simulink model "ExoskeletonControlModel"  (R2022b)
settings: Solver=ode3  StartTime=0.0  StopTime=inf  FixedStep=Ts  RelTol=1e-3
PreLoadFcn:
  | Ts_IO204 = 0.001;
  | 
  | if ~exist('Ts', 'var')
  | Ts = 0.001;
  | end
  | if ~exist('FPGA_Frequency', 'var')
  | FPGA_Frequency = 75000000;
  | end
  | 
  | ts_IO612 = 1e-3;
  | 
  | load('TargetReached.mat')
  | load('ActualPos_inc.mat')
model workspace (MAT data in the model file):
  DeltaData : timeseries (value not decoded)
  EC45_deg2incs = 2276
  EC60_deg2inc = 5461
  EC90_deg2incs = 7111
  Enc2rad_18bit = 2.3968e-05
  Enc2rad_19bit = 1.1984e-05
  Enc2rad_20bit = 5.9921e-06
  GiulioModel : robotics.RigidBodyTree (value not decoded)
  Giulio_Spheric_model : robotics.RigidBodyTree (value not decoded)
  Offset1_ticks = 571315
  Offset2_ticks = 590938.9928
  Offset3_ticks = 457912.8279
  Offset4_ticks = 482293.9763
  Offset5_ticks = 598735.9316
  Offset_M1 = 1.12645499896
  Offset_M2 = 4.02728553608
  Offset_M3 = 5.48587511336
  Offset_M4 = 2.03717511516
  Offset_M5 = 4.4996674016
  T1_Nm : object (value not decoded)
  T2_Nm : object (value not decoded)
  TBmodel : robotics.RigidBodyTree (value not decoded)
  Ts = 0.002
  Xg : object (value not decoded)
  Yg : object (value not decoded)
  Zg : object (value not decoded)
  a2 = 0.27
  change_variable = 0
  d1 = [0 0 0 0 0 0 0 0 0 0 0 0 ... (30001 elements, 30001x1)]
  d1_1 = 0.21074
  d2 = [0 0 0 0 0 0 0 0 0 0 0 0 ... (30001 elements, 30001x1)]
  d2_1 = 0.04864
  d3 = [0 0 0 0 0 0 0 0 0 0 0 0 ... (30001 elements, 30001x1)]
  d4 = [0 0 0 0 0 0 0 0 0 0 0 0 ... (30001 elements, 30001x1)]
  d5 = [0 0 0 0 0 0 0 0 0 0 0 0 ... (30001 elements, 30001x1)]
  d6 = [0 0 0 0 0 0 0 0 0 0 0 0 ... (30001 elements, 30001x1)]
  ee_x = -0.2852
  ee_y = -0.3683
  ee_z = -0.0386
  enc2rad_EC45 = 7.6699e-06
  enc2rad_EC90 = 2.3969e-05
  k1_Nm_ticks = 0.00923
  k2_Nm_ticks = 0.0257
  k3_Nm_ticks = 0.00692
  k4_Nm_ticks = 0.00729
  k5_Nm_ticks = 0.00641
  lower_lim_m1 = -330000
  lower_lim_m2 = -235302
  lower_lim_m3 = -132865
  lower_lim_m4 = -152732
  lower_lim_m5 = -138363
  lower_lim_m6 = -200325
  m1 = 2.441408578
  m2 = 3.750007
  m3 = 1.56250298
  m4 = 1.56250298
  m5 = 1.56250298
  m6 = 1.56250298
  n_oversampling = 8
  offset_sea_1 = 0.5547
  offset_sea_2 = 2.8595
  offset_sea_3 = 3.5058
  offset_sea_4 = 2.8586
  offset_sea_5 = 2.8736
  params : AKSIM (value not decoded)
  pos_th_neg = -180000
  pos_th_pos = 180000
  q1 = -1819347
  q2 = -196752
  q3 = -596465
  q4 = -556807
  q5 = -573932
  q6 = -489063
  sine = [0 0.187999937334 0.751998997352 1.69199492401 3.0079839574 4.6999608335 6.76791878442 9.21184953835 12.0317433196 15.2275888485 18.7993733417 22.7470825122 ... (12501 elements, 12501x1)]
  start : object (value not decoded)
  switch_admittance = 1
  t1 : object (value not decoded)
  t2 : object (value not decoded)
  torsionalStiffnes_M1 = 384.88
  torsionalStiffnes_M2 = 1500
  torsionalStiffnes_M3 = 901.97
  torsionalStiffnes_M4 = 950.86
  torsionalStiffnes_M5 = 930
  torsionalStiffnes_M6 = 914
  upper_lim_m1 = 340000
  upper_lim_m2 = 95467
  upper_lim_m3 = 164951
  upper_lim_m4 = 210607
  upper_lim_m5 = 252595
  upper_lim_m6 = 96694
  vel_th_neg = -100
  vel_th_pos = 100
  x = 0
undefined symbols (not defined in the file): C, DiscIntNeverNeededParam
libraries: canmsglib x285, speedgoatlib_IO614 x245, simulink x26, slrealtimeloglib x9, simulink_extras x6, robotmaniplib x6
(part 2 of 13)

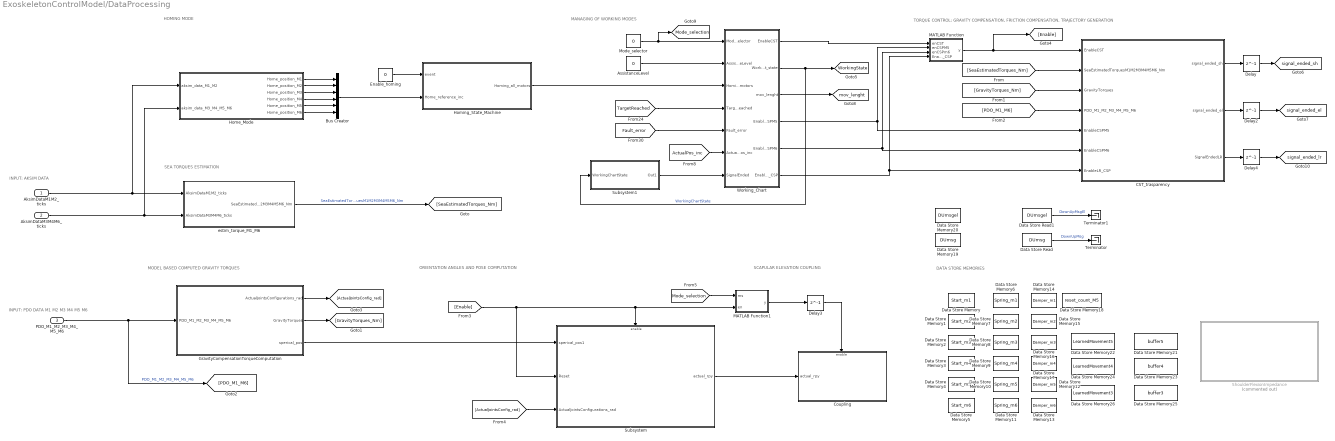
== system ExoskeletonControlModel/DataProcessing ==
  note: SCAPULAR ELEVATION COUPLING
  note: ORIENTATION ANGLES AND POSE COMPUTATION
  note: TORQUE CONTROL: GRAVITY COMPENSATION, FRICTION COMPENSATION, TRAJECTORY GENERATION
  note: MANAGING OF WORKING MODES
  note: DATA STORE MEMORIES
  note: INPUT: AKSIM DATA
  note: HOMING MODE
  note: MODEL BASED COMPUTED GRAVITY TORQUES
  note: INPUT: PDO DATA M1 M2 M3 M4 M5 M6
  note: SEA TORQUES ESTIMATION
  AksimDataM1M2_ticks : Inport
  AksimDataM3M4M6_ticks : Inport  Port=2
  PDO_M1_M2_M3_M4_M5_M6 : Inport  Port=3
  AssistanceLevel : Constant  Value=0
  Bus Creator : BusCreator  Inputs=6
  CST_trasparency : Subsystem
  Coupling : Subsystem
  Data Store Memory18 : DataStoreMemory  DataStoreName=reset_count_M5  ReadBeforeWriteMsg=warning  WriteAfterWriteMsg=warning  WriteAfterReadMsg=warning  ShowAdditionalParam=off  OutDataTypeStr=double
  Data Store Memory21 : DataStoreMemory  DataStoreName=buffer5  ReadBeforeWriteMsg=warning  WriteAfterWriteMsg=warning  WriteAfterReadMsg=warning  ShareAcrossModelInstances=on  VectorParams1D=off  ShowAdditionalParam=off  OutDataTypeStr=double  Dimensions=[10000,1]
  Data Store Memory22 : DataStoreMemory  DataStoreName=LearnedMovement5  ReadBeforeWriteMsg=warning  WriteAfterWriteMsg=warning  WriteAfterReadMsg=warning  ShareAcrossModelInstances=on  VectorParams1D=off  ShowAdditionalParam=off  OutDataTypeStr=double  Dimensions=[10000,1]
  Data Store Memory23 : DataStoreMemory  DataStoreName=buffer4  ReadBeforeWriteMsg=warning  WriteAfterWriteMsg=warning  WriteAfterReadMsg=warning  ShareAcrossModelInstances=on  VectorParams1D=off  ShowAdditionalParam=off  OutDataTypeStr=double  Dimensions=[10000,1]
  Data Store Memory24 : DataStoreMemory  DataStoreName=LearnedMovement4  ReadBeforeWriteMsg=warning  WriteAfterWriteMsg=warning  WriteAfterReadMsg=warning  ShareAcrossModelInstances=on  VectorParams1D=off  ShowAdditionalParam=off  OutDataTypeStr=double  Dimensions=[10000,1]
  Data Store Memory25 : DataStoreMemory  DataStoreName=buffer3  ReadBeforeWriteMsg=warning  WriteAfterWriteMsg=warning  WriteAfterReadMsg=warning  ShareAcrossModelInstances=on  VectorParams1D=off  ShowAdditionalParam=off  OutDataTypeStr=double  Dimensions=[10000,1]
  Data Store Memory26 : DataStoreMemory  DataStoreName=LearnedMovement3  ReadBeforeWriteMsg=warning  WriteAfterWriteMsg=warning  WriteAfterReadMsg=warning  ShareAcrossModelInstances=on  VectorParams1D=off  ShowAdditionalParam=off  OutDataTypeStr=double  Dimensions=[10000,1]
  Data Store Read : DataStoreRead  DataStoreName=DUmsg  IndexOptions=Index vector (dialog)  Indices=1  OutputSizes=1
  Data Store Read1 : DataStoreRead  DataStoreName=DUmsgel  IndexOptions=Index vector (dialog)  Indices=1  OutputSizes=1
  Data Store Memory : DataStoreMemory  DataStoreName=Start_m1  ReadBeforeWriteMsg=warning  WriteAfterWriteMsg=warning  WriteAfterReadMsg=warning  ShowAdditionalParam=off  OutDataTypeStr=double
  Data Store Memory1 : DataStoreMemory  DataStoreName=Start_m2  ReadBeforeWriteMsg=warning  WriteAfterWriteMsg=warning  WriteAfterReadMsg=warning  ShowAdditionalParam=off  OutDataTypeStr=double
  Data Store Memory10 : DataStoreMemory  DataStoreName=Spring_m5  ReadBeforeWriteMsg=warning  WriteAfterWriteMsg=warning  WriteAfterReadMsg=warning  ShowAdditionalParam=off  OutDataTypeStr=double
  Data Store Memory11 : DataStoreMemory  DataStoreName=Spring_m6  ReadBeforeWriteMsg=warning  WriteAfterWriteMsg=warning  WriteAfterReadMsg=warning  ShowAdditionalParam=off  OutDataTypeStr=double
  Data Store Memory12 : DataStoreMemory  DataStoreName=Damper_m5  ReadBeforeWriteMsg=warning  WriteAfterWriteMsg=warning  WriteAfterReadMsg=warning  ShowAdditionalParam=off  OutDataTypeStr=double
  Data Store Memory13 : DataStoreMemory  DataStoreName=Damper_m6  ReadBeforeWriteMsg=warning  WriteAfterWriteMsg=warning  WriteAfterReadMsg=warning  ShowAdditionalParam=off  OutDataTypeStr=double
  Data Store Memory14 : DataStoreMemory  DataStoreName=Damper_m1  ReadBeforeWriteMsg=warning  WriteAfterWriteMsg=warning  WriteAfterReadMsg=warning  ShowAdditionalParam=off  OutDataTypeStr=double
  Data Store Memory15 : DataStoreMemory  DataStoreName=Damper_m2  ReadBeforeWriteMsg=warning  WriteAfterWriteMsg=warning  WriteAfterReadMsg=warning  ShowAdditionalParam=off  OutDataTypeStr=double
  Data Store Memory16 : DataStoreMemory  DataStoreName=Damper_m3  ReadBeforeWriteMsg=warning  WriteAfterWriteMsg=warning  WriteAfterReadMsg=warning  ShowAdditionalParam=off  OutDataTypeStr=double
  Data Store Memory17 : DataStoreMemory  DataStoreName=Damper_m4  ReadBeforeWriteMsg=warning  WriteAfterWriteMsg=warning  WriteAfterReadMsg=warning  ShowAdditionalParam=off  OutDataTypeStr=double
  Data Store Memory19 : DataStoreMemory  DataStoreName=DUmsg  ReadBeforeWriteMsg=warning  WriteAfterWriteMsg=warning  WriteAfterReadMsg=warning  ShowAdditionalParam=off  OutDataTypeStr=double
  Data Store Memory2 : DataStoreMemory  DataStoreName=Start_m3  ReadBeforeWriteMsg=warning  WriteAfterWriteMsg=warning  WriteAfterReadMsg=warning  ShowAdditionalParam=off  OutDataTypeStr=double
  Data Store Memory20 : DataStoreMemory  DataStoreName=DUmsgel  ReadBeforeWriteMsg=warning  WriteAfterWriteMsg=warning  WriteAfterReadMsg=warning  ShowAdditionalParam=off  OutDataTypeStr=double
  Data Store Memory3 : DataStoreMemory  DataStoreName=Start_m4  ReadBeforeWriteMsg=warning  WriteAfterWriteMsg=warning  WriteAfterReadMsg=warning  ShowAdditionalParam=off  OutDataTypeStr=double
  Data Store Memory4 : DataStoreMemory  DataStoreName=Start_m5  ReadBeforeWriteMsg=warning  WriteAfterWriteMsg=warning  WriteAfterReadMsg=warning  ShowAdditionalParam=off  OutDataTypeStr=double
  Data Store Memory5 : DataStoreMemory  DataStoreName=Start_m6  ReadBeforeWriteMsg=warning  WriteAfterWriteMsg=warning  WriteAfterReadMsg=warning  ShowAdditionalParam=off  OutDataTypeStr=double
  Data Store Memory6 : DataStoreMemory  DataStoreName=Spring_m1  ReadBeforeWriteMsg=warning  WriteAfterWriteMsg=warning  WriteAfterReadMsg=warning  ShowAdditionalParam=off  OutDataTypeStr=double
  Data Store Memory7 : DataStoreMemory  DataStoreName=Spring_m2  ReadBeforeWriteMsg=warning  WriteAfterWriteMsg=warning  WriteAfterReadMsg=warning  ShowAdditionalParam=off  OutDataTypeStr=double
  Data Store Memory8 : DataStoreMemory  DataStoreName=Spring_m3  ReadBeforeWriteMsg=warning  WriteAfterWriteMsg=warning  WriteAfterReadMsg=warning  ShowAdditionalParam=off  OutDataTypeStr=double
  Data Store Memory9 : DataStoreMemory  DataStoreName=Spring_m4  ReadBeforeWriteMsg=warning  WriteAfterWriteMsg=warning  WriteAfterReadMsg=warning  ShowAdditionalParam=off  OutDataTypeStr=double
  Delay{,2..4} (4 alike) : Delay  DelayLength=1
  Enable_homing : Constant  Value=0
  GravityCompensationTorqueComputation : Subsystem
  Home_Mode : Subsystem
  Homing_State_Machine : Subsystem
  MATLAB Function : MATLAB Function  TreatAsAtomicUnit=on
  MATLAB Function1 : MATLAB Function  TreatAsAtomicUnit=on
  Mode_selector : Constant  Value=0
  ShoulderFlexionImpedance : Subsystem  Commented=on
  Subsystem : Subsystem
  Subsystem1 : Subsystem
  Terminator : Terminator
  Terminator1 : Terminator
  Working_Chart : Stateflow chart  TreatAsAtomicUnit=on
  estim_torque_M1_M6 : Subsystem
  tag scope: Mode_selection=global, WorkingState=global, mov_lenght=global, signal_ended_el=global, signal_ended_lr=global, signal_ended_sh=global
  wires:
  AksimDataM1M2_ticks/1 -> estim_torque_M1_M6/1(AksimDataM1M2_ticks), Home_Mode/1(aksim_data_M1_M2)
  AksimDataM3M4M6_ticks/1 -> Home_Mode/2(aksim_data_M3_M4_M5_M6), estim_torque_M1_M6/2(AksimDataM3M4M6_ticks)
  estim_torque_M1_M6/1(SeaEstimatedTorquesM1M2M3M4M5M6_Nm) -> [SeaEstimatedTorques_Nm]  "SeaEstimatedTorquesM1M2M3M4M5M6_Nm"
  Home_Mode/1(Home_position_M1) -> Bus Creator/1
  Home_Mode/2(Home_position_M2) -> Bus Creator/2
  Home_Mode/3(Home_position_M3) -> Bus Creator/3
  Home_Mode/4(Home_position_M4) -> Bus Creator/4
  Home_Mode/5(Home_position_M5) -> Bus Creator/5
  Bus Creator/1 -> Homing_State_Machine/2(Home_reference_inc)
  Home_Mode/6(Home_position_M6) -> Bus Creator/6
  GravityCompensationTorqueComputation/1(ActualJointsConfigurations_rad) -> [ActualJointsConfig_rad]
  GravityCompensationTorqueComputation/2(GravityTorques) -> [GravityTorques_Nm]
  GravityCompensationTorqueComputation/3(sperical_pos) -> Subsystem/1(sperical_pos1)
  Subsystem/1(actual_rpy) -> Coupling/1(actual_rpy)
  [Enable] -> Subsystem/2(Reset), Subsystem/Enable, MATLAB Function1/2(en)
  PDO_M1_M2_M3_M4_M5_M6/1 -> [PDO_M1_M6], GravityCompensationTorqueComputation/1(PDO_M1_M2_M3_M4_M5_M6)  "PDO_M1_M2_M3_M4_M5_M6"
  Enable_homing/1 -> Homing_State_Machine/1(event)
  Mode_selector/1 -> [Mode_selection], Working_Chart/1(Mode_selector)
  Homing_State_Machine/1(Homing_all_motors) -> Working_Chart/3(Homing_all_motors)
  Working_Chart/1(EnableCST) -> MATLAB Function/1(enCST)
  [SeaEstimatedTorques_Nm] -> CST_trasparency/2(SeaEstimatedTorquesM1M2M3M4M5M6_Nm)
  [GravityTorques_Nm] -> CST_trasparency/3(GravityTorques)
  [PDO_M1_M6] -> CST_trasparency/4(PDO_M1_M2_M3_M4_M5_M6)
  [TargetReached] -> Working_Chart/4(TargetReached)
  Working_Chart/2(Working_Chart_state) -> Subsystem1/1(WorkingChartState), [WorkingState]  "WorkingChartState"
  [ActualJointsConfig_rad] -> Subsystem/3(ActualJointsConfigurations_rad)
  [Fault_error] -> Working_Chart/5(Fault_error)
  CST_trasparency/1(signal_ended_sh) -> Delay/1
  Delay/1 -> [signal_ended_sh]
  Delay2/1 -> [signal_ended_el]
  CST_trasparency/2(signal_ended_el) -> Delay2/1
  Delay3/1 -> Coupling/Enable
  [ActualPos_inc] -> Working_Chart/6(ActualPos_inc)
  Working_Chart/3(mov_lenght) -> [mov_lenght]
  Delay4/1 -> [signal_ended_lr]
  CST_trasparency/3(SignalEndedLR) -> Delay4/1
  Subsystem1/1(Out1) -> Working_Chart/7(SignalEnded)
  AssistanceLevel/1 -> Working_Chart/2(AssistanceLevel)
  Working_Chart/4(EnableCSPM5) -> CST_trasparency/5(EnableCSPM5), MATLAB Function/2(enCSPM5)
  Working_Chart/5(EnableCSPM6) -> CST_trasparency/6(EnableCSPM6), MATLAB Function/3(enCSPm6)
  MATLAB Function/1(y) -> [Enable], CST_trasparency/1(EnableCST)
  MATLAB Function1/1(y) -> Delay3/1
  [Mode_selection] -> MATLAB Function1/1(ms)
  Working_Chart/6(EnableLR_CSP) -> CST_trasparency/7(EnableLR_CSP), MATLAB Function/4(EnableLR_CSP)
  Data Store Read/1 -> Terminator/1  "DownUpMsg"
  Data Store Read1/1 -> Terminator1/1  "DownUpMsgEl"

== system ExoskeletonControlModel/InputDataRX ==
  note: PDO M1 M2 M3 M4 M5
  note: EPOS M3-M4-M5-M6 - CAN MSG
  note: EPOS M1-M2 - CAN MSG
  note: FROM TIVA - ENCODERS - CAN MSG
  note: DATA TO BE PROCESSED
  Bus Creator : BusCreator  Inputs=6
  Bus Creator1 : BusCreator  Inputs=3
  Bus Creator2 : BusCreator  Inputs=3
  CAN Read Loop - Channel 1 - M1-M2 : Subsystem  TreatAsAtomicUnit=on
  CAN Read Loop - Channel 2 - M3-M5 : Subsystem  TreatAsAtomicUnit=on
  CAN Read Loop - Channel 3 : Subsystem  TreatAsAtomicUnit=on
  CAN Read Loop - Channel 4 : Subsystem  TreatAsAtomicUnit=on
  PDOm1m6 : slrealtimeloglib/File Log  decimation=1  inputProcessing=Elements as channels (sample based)
  RX Sample Time : Constant  SampleTime=Ts
  Terminator : Terminator
  Terminator4 : Terminator
  AksimDataM1M2_ticks : Outport
  AksimDataM3M4M6_ticks : Outport  Port=2
  PDO_M1_M2_M3_M4_M5_M6 : Outport  Port=3
  tag scope: AksimDataM1_M2=global, AksimDataM3_M6=global, PDO_M1_M6=global, stat_mode_nmt_M1_M2=global, stat_mode_nmt_M3_M5_M6=global
  wires:
  CAN Read Loop - Channel 2 - M3-M5/1(aksim_data_M3_M5) -> [AksimDataM3_M6]
  CAN Read Loop - Channel 1 - M1-M2/1(aksim_data_M1_M2) -> [AksimDataM1_M2]
  RX Sample Time/1 -> CAN Read Loop - Channel 4/1(SampleTime), CAN Read Loop - Channel 2 - M3-M5/1(SampleTime), CAN Read Loop - Channel 3/1(SampleTime), CAN Read Loop - Channel 1 - M1-M2/1(SampleTime)
  CAN Read Loop - Channel 3/1(SDOs) -> Terminator/1
  CAN Read Loop - Channel 3/2(emcy) -> Bus Creator1/1  "emcy_M1_M2"
  CAN Read Loop - Channel 3/3(NMT_state) -> Bus Creator1/2  "NMT_state_M1_M2"
  CAN Read Loop - Channel 3/4(status_mode_m1_m2) -> Bus Creator1/3  "status_mode_M1_M2"
  CAN Read Loop - Channel 4/1(SDOs) -> Terminator4/1
  CAN Read Loop - Channel 4/2(emcy) -> Bus Creator2/1  "emcy"
  CAN Read Loop - Channel 4/3(NMT_state) -> Bus Creator2/2  "NMT_state"
  CAN Read Loop - Channel 4/4(status_mode_m3_m4_m5_m6) -> Bus Creator2/3
  CAN Read Loop - Channel 4/7(PDO_m5) -> [PDO_m5]  "PDO_M5"
  CAN Read Loop - Channel 4/6(PDO_m4) -> [PDO_m4]  "PDO_M4"
  CAN Read Loop - Channel 4/5(PDO_m3) -> [PDO_m3]  "PDO_M3"
  Bus Creator/1 -> PDOm1m6/1, [PDO_M1_M6]
  Bus Creator1/1 -> [stat_mode_nmt_M1_M2]
  Bus Creator2/1 -> [stat_mode_nmt_M3_M5_M6]
  [PDO_m1] -> Bus Creator/1  "PDO_M1"
  CAN Read Loop - Channel 3/5(PDO_m1) -> [PDO_m1]  "PDO_M1"
  CAN Read Loop - Channel 3/6(PDO_m2) -> [PDO_m2]  "PDO_M2"
  [PDO_m2] -> Bus Creator/2  "PDO_M2"
  [PDO_m3] -> Bus Creator/3  "PDO_M3"
  [PDO_m4] -> Bus Creator/4  "PDO_M4"
  [PDO_m5] -> Bus Creator/5  "PDO_M5"
  [AksimDataM1_M2] -> AksimDataM1M2_ticks/1
  [AksimDataM3_M6] -> AksimDataM3M4M6_ticks/1
  [PDO_M1_M6] -> PDO_M1_M2_M3_M4_M5_M6/1
  CAN Read Loop - Channel 4/8(PDO_m6) -> [PDO_m6]
  [PDO_m6] -> Bus Creator/6  "PDO_M6"

== system ExoskeletonControlModel/OutputDataTX ==
  SendPositionToEPOS : Subsystem  Commented=on
  TX_EPOS4_M1_M2 : Subsystem
  TX_EPOS4_M3_M5 : Subsystem

== system ExoskeletonControlModel/DataProcessing/CST_trasparency ==
  note: CURRENT/TORQUE CONTROL
  note: SEA ESTIMATED TORQUES Nm
  EnableCST : Inport
  SeaEstimatedTorquesM1M2M3M4M5M6_Nm : Inport  Port=2
  GravityTorques : Inport  Port=3
  PDO_M1_M2_M3_M4_M5_M6 : Inport  Port=4
  EnableCSPM5 : Inport  Port=5
  EnableCSPM6 : Inport  Port=6
  EnableLR_CSP : Inport  Port=7
  CST_control : Subsystem
  Data Store Write : DataStoreWrite  DataStoreName=DUmsg  IndexOptions=Index vector (dialog)  Indices=1  OutputSizes=1
  Data Store Write1 : DataStoreWrite  DataStoreName=DUmsgel  IndexOptions=Index vector (dialog)  Indices=1  OutputSizes=1
  Delay{,2..4} (4 alike) : Delay  DelayLength=1
  Delay1 : Delay  DelayLength=3
  Demux1 : Demux  Outputs=6
  Gain : Gain
  Gain1 : Gain
  Mux : Mux  Inputs=3
  Repetition : Constant
  SendTorqueCommand : Subsystem
  Terminator : Terminator
  duration : Constant  Value=10
  max : Constant  Value=60
  signal_ended_sh : Outport
  signal_ended_el : Outport  Port=2
  SignalEndedLR : Outport  Port=3
  wires:
  CST_control/1(Ref Drive Torque - Motor6) -> SendTorqueCommand/2(TAU_M6)  "target_torque_m6"
  EnableCST/1 -> CST_control/Enable, Delay1/1, Delay/1
  CST_control/2(Ref Drive Torque - Motor5) -> SendTorqueCommand/3(TAU_M5)
  CST_control/3(Ref Drive Torque - Motor4) -> SendTorqueCommand/4(TAU_M4)
  CST_control/4(Ref Drive Torque - Motor3) -> SendTorqueCommand/5(TAU_M3)
  GravityTorques/1 -> CST_control/3(GravityTorques)
  PDO_M1_M2_M3_M4_M5_M6/1 -> CST_control/4(PDO_M1_M2_M3_M4_M5_M6)
  Delay/1 -> CST_control/1(enable_signal)
  Delay1/1 -> SendTorqueCommand/1(In1)
  CST_control/5(signal_ended_sh) -> signal_ended_sh/1
  [WorkingState] -> CST_control/5(State)
  CST_control/6(signal_ended_el) -> signal_ended_el/1
  [mov_lenght] -> CST_control/6(MovLenght)
  [Mode_selection] -> CST_control/7(ModeSelection)
  CST_control/7(SignalEndedLR) -> SignalEndedLR/1
  EnableCSPM5/1 -> Delay2/1
  EnableCSPM6/1 -> Delay3/1
  Delay2/1 -> CST_control/8(EnableCSPM5)
  Delay3/1 -> CST_control/9(EnableCSPM6)
  Demux1/3 -> [SeaEstimatedTorqueM3_Nm]
  Demux1/5 -> [SeaEstimatedTorqueM5_Nm]
  Demux1/6 -> [SeaEstimatedTorqueM6_Nm]
  Demux1/4 -> [SeaEstimatedTorqueM4_Nm]
  Demux1/1 -> [SeaEstimatedTorqueM1_Nm]  "SeaEstimatedTorqueM1_Nm"
  Demux1/2 -> [SeaEstimatedTorqueM2_Nm]
  SeaEstimatedTorquesM1M2M3M4M5M6_Nm/1 -> Demux1/1, CST_control/2(Measured SEA torque | Nm)
  [SeaEstimatedTorqueM1_Nm] -> SendTorqueCommand/6(In6)
  EnableLR_CSP/1 -> Delay4/1
  Delay4/1 -> CST_control/10(EnableLR)
  duration/1 -> Mux/3
  Repetition/1 -> Mux/2
  Mux/1 -> CST_control/11(MovSet)
  max/1 -> Mux/1
  CST_control/8(updownM5) -> Gain/1
  Gain/1 -> Data Store Write/1, Terminator/1  "udsignal"
  CST_control/9(updownM6) -> Gain1/1
  Gain1/1 -> Data Store Write1/1  "udsignalel"

== system ExoskeletonControlModel/DataProcessing/Coupling ==
  actual_rpy : Inport
  Enable : EnablePort
  Constant : Constant  Value=4
  Constant1 : Constant  Value=0
  Constant2 : Constant  Value=60
  Demux : Demux  Outputs=3
  Divide : Product  Inputs=*/
  Gain : Gain  Gain=-1
  Gain11 : Gain  Gain=EC60_deg2inc
  Round1 : Rounding  Operator=round
  Sum : Sum  Inputs=|++
  Switch : Switch  Criteria=u2 > Threshold  SaturateOnIntegerOverflow=off  InputSameDT=off
  Terminator : Terminator
  Terminator1 : Terminator
  receive_PDO3_m2 : Subsystem
  stauration_2 : Saturate  UpperLimit=106389-(2*5461)  LowerLimit=-246224+(2*5461)
  wires:
  Round1/1 -> Gain/1
  Gain11/1 -> Round1/1
  stauration_2/1 -> receive_PDO3_m2/1(target_pos)
  Demux/1 -> Terminator/1
  Demux/3 -> Terminator1/1
  actual_rpy/1 -> Demux/1
  Divide/1 -> Gain11/1
  Constant/1 -> Divide/2
  Switch/1 -> Divide/1
  Constant1/1 -> Switch/3
  Gain/1 -> stauration_2/1
  Demux/2 -> Sum/1  "p"
  Sum/1 -> Switch/1, Switch/2
  Constant2/1 -> Sum/2

== system ExoskeletonControlModel/DataProcessing/GravityCompensationTorqueComputation ==
  note: CONVERSION TICKS TO DEG
  PDO_M1_M2_M3_M4_M5_M6 : Inport
  Bus Creator : BusCreator  Inputs=6  OutDataTypeStr=Bus: ActualPos_inc
  Bus Selector1 : BusSelector  OutputSignals=PDO_M1.pos_actual_1,PDO_M2.pos_actual_2,PDO_M3.pos_actual_3,PDO_M4.pos_actual_4,PDO_M5.pos_actual_5,PDO_M6.pos_actual_6
  Bus Selector5 : BusSelector  OutputSignals=PDO_M1.pos_actual_1,PDO_M2.pos_actual_2,PDO_M3.pos_actual_3,PDO_M4.pos_actual_4,PDO_M5.pos_actual_5,PDO_M6.pos_actual_6
  Degrees to Radians1 : simulink_extras/Transformations/Degrees to Radians
  Degrees to Radians5 : simulink_extras/Transformations/Degrees to Radians
  Gain{7..9,18} (4 alike) : Gain  Gain=1/EC45_deg2incs
  Gain5 : Gain  Gain=1/EC90_deg2incs
  Gain6 : Gain  Gain=1/EC60_deg2inc
  Gravity Torque : robotmaniplib/Gravity Torque  RigidBodyTree=GiulioModel  SimulateUsing=Interpreted execution
  Joints_degrees : Subsystem
  ModelBasedGravityTorques : slrealtimeloglib/File Log  decimation=1  inputProcessing=Elements as channels (sample based)
  Mux : Mux  Inputs=3
  Mux4 : Mux  Inputs=6
  ActualJointsConfigurations_rad : Outport
  GravityTorques : Outport  Port=2
  sperical_pos : Outport  Port=3
  tag scope: ActualPos_inc=global
  wires:
  Bus Selector5/4 -> Gain8/1  "<pos_actual_4>"
  Bus Selector5/1 -> Gain5/1  "<pos_actual_1>"
  Bus Selector5/6 -> Gain18/1  "<pos_actual_6>"
  Gain7/1 -> Mux/1, Mux4/3
  Bus Selector5/5 -> Gain9/1  "<pos_actual_5>"
  Gain8/1 -> Mux/2, Mux4/4
  Bus Selector5/2 -> Gain6/1  "<pos_actual_2>"
  Bus Selector5/3 -> Gain7/1  "<pos_actual_3>"
  Gain6/1 -> Mux4/2
  Degrees to Radians5/1 -> Gravity Torque/1, ActualJointsConfigurations_rad/1  "ActualJointsConfigurations_rad"
  Gain9/1 -> Mux/3, Mux4/5
  Gain5/1 -> Mux4/1
  Mux4/1 -> Degrees to Radians5/1
  Gain18/1 -> Mux4/6
  Gravity Torque/1 -> ModelBasedGravityTorques/1, GravityTorques/1
  Mux/1 -> Degrees to Radians1/1
  Degrees to Radians1/1 -> sperical_pos/1
  Bus Selector1/6 -> Bus Creator/6  "<pos_actual_6>"
  PDO_M1_M2_M3_M4_M5_M6/1 -> Bus Selector1/1, Bus Selector5/1, Joints_degrees/1(PDO_M1_M2_M3_M4_M5_M6)
  Bus Selector1/2 -> Bus Creator/2  "<pos_actual_2>"
  Bus Selector1/5 -> Bus Creator/5  "<pos_actual_5>"
  Bus Selector1/3 -> Bus Creator/3  "<pos_actual_3>"
  Bus Selector1/1 -> Bus Creator/1  "<pos_actual_1>"
  Bus Selector1/4 -> Bus Creator/4  "<pos_actual_4>"
  Bus Creator/1 -> [ActualPos_inc]

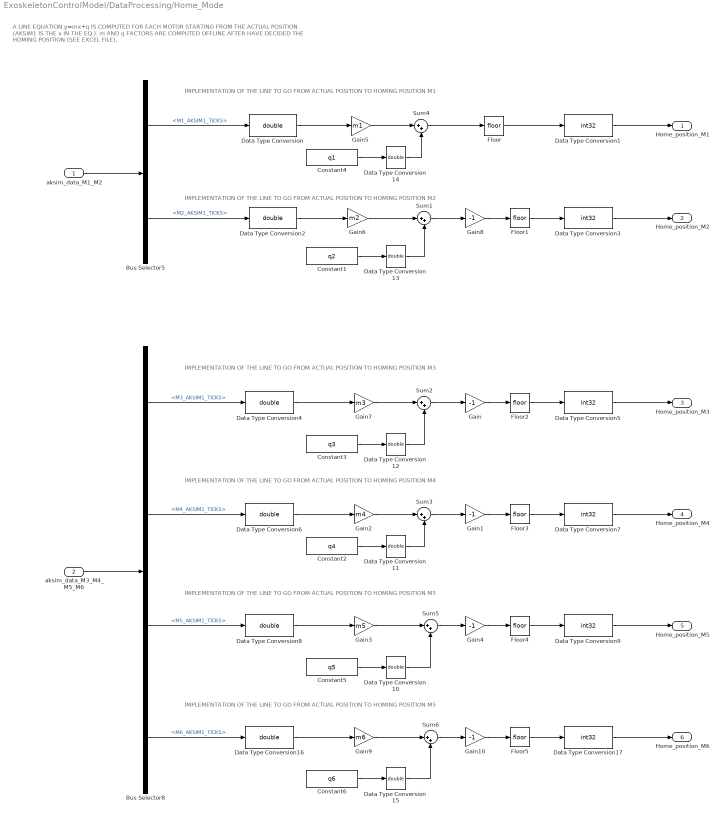
== system ExoskeletonControlModel/DataProcessing/Home_Mode ==
  note: A LINE EQUATION y=mx+q IS COMPUTED FOR EACH MOTOR STARTING FROM THE ACTUAL POSITION (AKSIM1 IS THE x IN THE EQ.).
      | m AND q FACTORS ARE COMPUTED OFFLINE AFTER HAVE DECIDED THE HOMING POSITION (SEE EXCEL FILE).
  note: IMPLEMENTATION OF THE LINE TO GO FROM ACTUAL POSITION TO HOMING POSITION M1
  note: IMPLEMENTATION OF THE LINE TO GO FROM ACTUAL POSITION TO HOMING POSITION M2
  note: IMPLEMENTATION OF THE LINE TO GO FROM ACTUAL POSITION TO HOMING POSITION M3
  note: IMPLEMENTATION OF THE LINE TO GO FROM ACTUAL POSITION TO HOMING POSITION M4
  note: IMPLEMENTATION OF THE LINE TO GO FROM ACTUAL POSITION TO HOMING POSITION M5
  note: IMPLEMENTATION OF THE LINE TO GO FROM ACTUAL POSITION TO HOMING POSITION M5
  aksim_data_M1_M2 : Inport
  aksim_data_M3_M4_M5_M6 : Inport  Port=2
  Bus Selector5 : BusSelector  OutputSignals=M1_TICKS.M1_AKSIM1_TICKS,M2_TICKS.M2_AKSIM1_TICKS
  Bus Selector8 : BusSelector  OutputSignals=M3_TICKS.M3_AKSIM1_TICKS,M4_TICKS.M4_AKSIM1_TICKS,M5_TICKS.M5_AKSIM1_TICKS,M6_TICKS.M6_AKSIM1_TICKS
  Constant1 : Constant  Value=q2  OutDataTypeStr=double
  Constant2 : Constant  Value=q4  OutDataTypeStr=double
  Constant3 : Constant  Value=q3  OutDataTypeStr=double
  Constant4 : Constant  Value=q1  OutDataTypeStr=double
  Constant5 : Constant  Value=q5  OutDataTypeStr=double
  Constant6 : Constant  Value=q6  OutDataTypeStr=double
  Data Type Conversion{,2,4,6,8,10..16} (12 alike) : DataTypeConversion  OutDataTypeStr=double  SaturateOnIntegerOverflow=off  RndMeth=Floor
  Data Type Conversion{1,3,5,7,9,17} (6 alike) : DataTypeConversion  OutDataTypeStr=int32  SaturateOnIntegerOverflow=off  RndMeth=Floor
  Floor{,1..5} (6 alike) : Rounding
  Gain{,1,4,8,10} (5 alike) : Gain  Gain=-1
  Gain2 : Gain  Gain=m4  ParamDataTypeStr=double  OutDataTypeStr=double
  Gain3 : Gain  Gain=m5  ParamDataTypeStr=double  OutDataTypeStr=double
  Gain5 : Gain  Gain=m1  ParamDataTypeStr=double  OutDataTypeStr=double
  Gain6 : Gain  Gain=m2  ParamDataTypeStr=double  OutDataTypeStr=double
  Gain7 : Gain  Gain=m3  ParamDataTypeStr=double  OutDataTypeStr=double
  Gain9 : Gain  Gain=m6  ParamDataTypeStr=double  OutDataTypeStr=double
  Sum{1..6} (6 alike) : Sum  Inputs=|++
  Home_position_M1 : Outport
  Home_position_M2 : Outport  Port=2
  Home_position_M3 : Outport  Port=3
  Home_position_M4 : Outport  Port=4
  Home_position_M5 : Outport  Port=5
  Home_position_M6 : Outport  Port=6
  wires:
  Bus Selector5/1 -> Data Type Conversion/1  "<M1_AKSIM1_TICKS>"
  Floor1/1 -> Data Type Conversion3/1
  Floor3/1 -> Data Type Conversion7/1
  Sum5/1 -> Gain4/1
  Bus Selector5/2 -> Data Type Conversion2/1  "<M2_AKSIM1_TICKS>"
  Bus Selector8/3 -> Data Type Conversion8/1  "<M5_AKSIM1_TICKS>"
  Sum1/1 -> Gain8/1
  Bus Selector8/2 -> Data Type Conversion6/1  "<M4_AKSIM1_TICKS>"
  Floor2/1 -> Data Type Conversion5/1
  Floor4/1 -> Data Type Conversion9/1
  Bus Selector8/1 -> Data Type Conversion4/1  "<M3_AKSIM1_TICKS>"
  Sum2/1 -> Gain/1
  aksim_data_M1_M2/1 -> Bus Selector5/1
  Floor/1 -> Data Type Conversion1/1
  Sum3/1 -> Gain1/1
  aksim_data_M3_M4_M5_M6/1 -> Bus Selector8/1
  Constant5/1 -> Data Type Conversion10/1
  Data Type Conversion10/1 -> Sum5/2
  Data Type Conversion6/1 -> Gain2/1
  Data Type Conversion11/1 -> Sum3/2
  Constant2/1 -> Data Type Conversion11/1
  Data Type Conversion4/1 -> Gain7/1
  Data Type Conversion12/1 -> Sum2/2
  Constant3/1 -> Data Type Conversion12/1
  Data Type Conversion2/1 -> Gain6/1
  Constant1/1 -> Data Type Conversion13/1
  Data Type Conversion13/1 -> Sum1/2
  Sum4/1 -> Floor/1
  Data Type Conversion/1 -> Gain5/1
  Data Type Conversion14/1 -> Sum4/2
  Constant4/1 -> Data Type Conversion14/1
  Gain5/1 -> Sum4/1
  Gain6/1 -> Sum1/1
  Gain7/1 -> Sum2/1
  Gain2/1 -> Sum3/1
  Data Type Conversion8/1 -> Gain3/1
  Gain3/1 -> Sum5/1
  Gain/1 -> Floor2/1
  Gain1/1 -> Floor3/1
  Gain4/1 -> Floor4/1
  Gain8/1 -> Floor1/1
  Data Type Conversion1/1 -> Home_position_M1/1
  Data Type Conversion3/1 -> Home_position_M2/1
  Data Type Conversion5/1 -> Home_position_M3/1
  Data Type Conversion7/1 -> Home_position_M4/1
  Data Type Conversion9/1 -> Home_position_M5/1
  Data Type Conversion17/1 -> Home_position_M6/1
  Gain9/1 -> Sum6/1
  Gain10/1 -> Floor5/1
  Data Type Conversion16/1 -> Gain9/1
  Constant6/1 -> Data Type Conversion15/1
  Data Type Conversion15/1 -> Sum6/2
  Floor5/1 -> Data Type Conversion17/1
  Sum6/1 -> Gain10/1
  Bus Selector8/4 -> Data Type Conversion16/1  "<M6_AKSIM1_TICKS>"

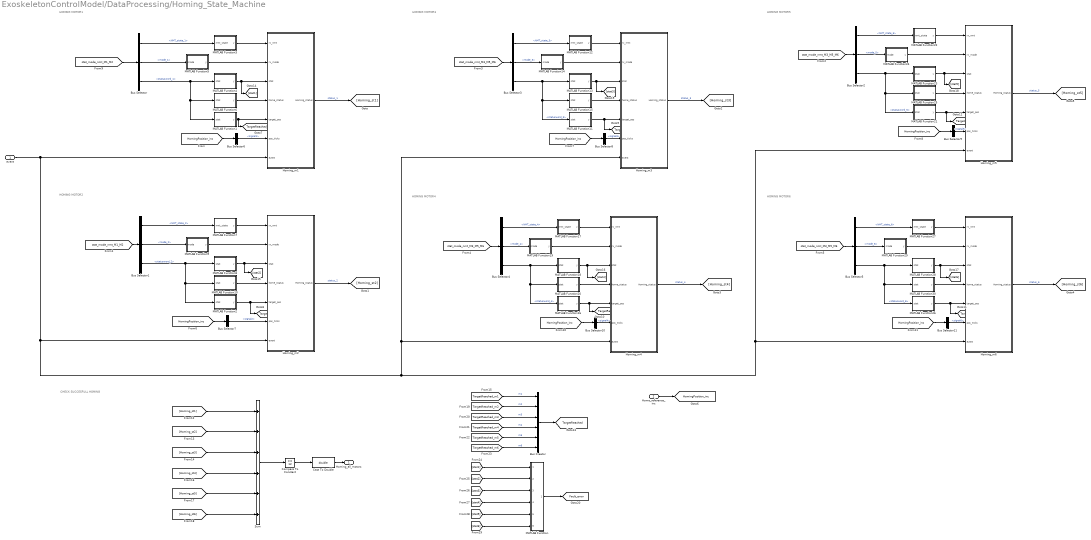
== system ExoskeletonControlModel/DataProcessing/Homing_State_Machine ==
  note: CHECK SUCCESFULL HOMING
  note: HOMING MOTOR1
  note: HOMING MOTOR2
  note: HOMING MOTOR3
  note: HOMING MOTOR5
  note: HOMING MOTOR6
  note: HOMING MOTOR4
  event : Inport
  Home_reference_inc : Inport  Port=2
  Bus Creator : BusCreator  Inputs=6  OutDataTypeStr=Bus: TargetReached
  Bus Selector : BusSelector  OutputSignals=NMT_state_M1_M2.NMT_state_1,status_mode_M1_M2.mode_1,status_mode_M1_M2.statusword_1
  Bus Selector1 : BusSelector  OutputSignals=NMT_state_M1_M2.NMT_state_2,status_mode_M1_M2.mode_2,status_mode_M1_M2.statusword_2
  Bus Selector10 : BusSelector  OutputSignals=signal4
  Bus Selector11 : BusSelector  OutputSignals=signal6
  Bus Selector2 : BusSelector  OutputSignals=NMT_state.NMT_state_5,signal3.mode_5,signal3.statusword_5
  Bus Selector3 : BusSelector  OutputSignals=NMT_state.NMT_state_3,signal3.mode_3,signal3.statusword_3
  Bus Selector4 : BusSelector  OutputSignals=NMT_state.NMT_state_4,signal3.mode_4,signal3.statusword_4
  Bus Selector5 : BusSelector  OutputSignals=NMT_state.NMT_state_6,signal3.mode_6,signal3.statusword_6
  Bus Selector6 : BusSelector  OutputSignals=signal1
  Bus Selector7 : BusSelector  OutputSignals=signal2
  Bus Selector8 : BusSelector  OutputSignals=signal3
  Bus Selector9 : BusSelector  OutputSignals=signal5
  Cast To Double : DataTypeConversion  OutDataTypeStr=double  SaturateOnIntegerOverflow=off  RndMeth=Floor
  Compare To Constant : simulink/Logic and Bit Operations/Compare To Constant  relop===  const=12  OutDataTypeStr=uint8
  Homing_m1 : Stateflow chart  TreatAsAtomicUnit=on
  Homing_m2 : Stateflow chart  TreatAsAtomicUnit=on
  Homing_m3 : Stateflow chart  TreatAsAtomicUnit=on
  Homing_m4 : Stateflow chart  TreatAsAtomicUnit=on
  Homing_m5 : Stateflow chart  TreatAsAtomicUnit=on
  Homing_m6 : Stateflow chart  TreatAsAtomicUnit=on
  MATLAB Function : MATLAB Function  TreatAsAtomicUnit=on
  MATLAB Function1 : MATLAB Function  TreatAsAtomicUnit=on
  MATLAB Function10 : MATLAB Function  TreatAsAtomicUnit=on
  MATLAB Function11 : MATLAB Function  TreatAsAtomicUnit=on
  MATLAB Function12 : MATLAB Function  TreatAsAtomicUnit=on
  MATLAB Function13 : MATLAB Function  TreatAsAtomicUnit=on
  MATLAB Function14 : MATLAB Function  TreatAsAtomicUnit=on
  MATLAB Function15 : MATLAB Function  TreatAsAtomicUnit=on
  MATLAB Function16 : MATLAB Function  TreatAsAtomicUnit=on
  MATLAB Function17 : MATLAB Function  TreatAsAtomicUnit=on
  MATLAB Function18 : MATLAB Function  TreatAsAtomicUnit=on
  MATLAB Function19 : MATLAB Function  TreatAsAtomicUnit=on
  MATLAB Function2 : MATLAB Function  TreatAsAtomicUnit=on
  MATLAB Function20 : MATLAB Function  TreatAsAtomicUnit=on
  MATLAB Function21 : MATLAB Function  TreatAsAtomicUnit=on
  MATLAB Function22 : MATLAB Function  TreatAsAtomicUnit=on
  MATLAB Function23 : MATLAB Function  TreatAsAtomicUnit=on
  MATLAB Function24 : MATLAB Function  TreatAsAtomicUnit=on
  MATLAB Function25 : MATLAB Function  TreatAsAtomicUnit=on
  MATLAB Function26 : MATLAB Function  TreatAsAtomicUnit=on
  MATLAB Function27 : MATLAB Function  TreatAsAtomicUnit=on
  MATLAB Function28 : MATLAB Function  TreatAsAtomicUnit=on
  MATLAB Function29 : MATLAB Function  TreatAsAtomicUnit=on
  MATLAB Function3 : MATLAB Function  TreatAsAtomicUnit=on
  MATLAB Function30 : MATLAB Function  TreatAsAtomicUnit=on
  MATLAB Function4 : MATLAB Function  TreatAsAtomicUnit=on
  MATLAB Function5 : MATLAB Function  TreatAsAtomicUnit=on
  MATLAB Function6 : MATLAB Function  TreatAsAtomicUnit=on
  MATLAB Function7 : MATLAB Function  TreatAsAtomicUnit=on
  MATLAB Function8 : MATLAB Function  TreatAsAtomicUnit=on
  MATLAB Function9 : MATLAB Function  TreatAsAtomicUnit=on
  Sum : Sum  Inputs=++++++
  Homing_all_motors : Outport
  tag scope: Fault_error=global, HomingPosition_inc=global, TargetReached=global, TargetReached_m1=global, TargetReached_m2=global, TargetReached_m3=global, TargetReached_m4=global, TargetReached_m5=global, TargetReached_m6=global
  wires:
  MATLAB Function24/1(y) -> Homing_m5/2(rx_mode)
  MATLAB Function10/1(y) -> Homing_m2/4(home_status)
  MATLAB Function25/1(y) -> Homing_m5/4(home_status)
  MATLAB Function16/1(y) -> [TargetReached_m4], Homing_m4/5(target_pos)
  Bus Selector2/3 -> MATLAB Function21/1(stat), MATLAB Function25/1(stat), MATLAB Function23/1(stat)  "<statusword_5>"
  Bus Selector5/3 -> MATLAB Function28/1(stat), MATLAB Function30/1(stat), MATLAB Function26/1(stat)  "<statusword_6>"
  Bus Selector/1 -> MATLAB Function3/1(nmt_state)  "<NMT_state_1>"
  MATLAB Function20/1(y) -> Homing_m4/4(home_status)
  [HomingPosition_inc] -> Bus Selector10/1
  MATLAB Function18/1(y) -> [stat4], Homing_m4/3(stat)
  MATLAB Function4/1(y) -> Homing_m1/3(stat), [stat1]
  [HomingPosition_inc] -> Bus Selector8/1
  MATLAB Function21/1(y) -> [TargetReached_m5], Homing_m5/5(target_pos)
  event/1 -> Homing_m1/7(event), Homing_m3/7(event), Homing_m4/7(event), Homing_m6/7(event), Homing_m5/7(event), Homing_m2/7(event)
  Bus Selector6/1 -> Homing_m1/6(pos_ticks)  "<signal1>"
  MATLAB Function22/1(y) -> Homing_m5/1(rx_nmt)
  Bus Selector4/3 -> MATLAB Function18/1(stat), MATLAB Function16/1(stat), MATLAB Function20/1(stat)  "<statusword_4>"
  Bus Selector1/3 -> MATLAB Function8/1(stat), MATLAB Function2/1(stat), MATLAB Function10/1(stat)  "<statusword_2>"
  Bus Selector10/1 -> Homing_m4/6(pos_ticks)  "<signal4>"
  MATLAB Function26/1(y) -> [TargetReached_m6], Homing_m6/5(target_pos)
  Bus Selector8/1 -> Homing_m3/6(pos_ticks)  "<signal3>"
  MATLAB Function6/1(y) -> Homing_m1/4(home_status)
  Bus Selector3/3 -> MATLAB Function13/1(stat), MATLAB Function11/1(stat), MATLAB Function15/1(stat)  "<statusword_3>"
  MATLAB Function29/1(y) -> Homing_m6/2(rx_mode)
  [stat_mode_nmt_M1_M2] -> Bus Selector/1
  Bus Selector1/1 -> MATLAB Function7/1(nmt_state)  "<NMT_state_2>"
  Bus Selector2/1 -> MATLAB Function22/1(nmt_state)  "<NMT_state_5>"
  MATLAB Function5/1(y) -> Homing_m1/2(rx_mode)
  MATLAB Function17/1(y) -> Homing_m4/1(rx_nmt)
  MATLAB Function27/1(y) -> Homing_m6/1(rx_nmt)
  [HomingPosition_inc] -> Bus Selector11/1
  MATLAB Function28/1(y) -> [stat6], Homing_m6/3(stat)
  MATLAB Function30/1(y) -> Homing_m6/4(home_status)
  MATLAB Function1/1(y) -> [TargetReached_m1], Homing_m1/5(target_pos)
  MATLAB Function7/1(y) -> Homing_m2/1(rx_nmt)
  Bus Selector/3 -> MATLAB Function6/1(stat), MATLAB Function1/1(stat), MATLAB Function4/1(stat)  "<statusword_1>"
  MATLAB Function23/1(y) -> [stat5], Homing_m5/3(stat)
  MATLAB Function11/1(y) -> [TargetReached_m3], Homing_m3/5(target_pos)
  [stat_mode_nmt_M1_M2] -> Bus Selector1/1
  Bus Selector9/1 -> Homing_m5/6(pos_ticks)  "<signal5>"
  MATLAB Function12/1(y) -> Homing_m3/1(rx_nmt)
  [stat_mode_nmt_M3_M5_M6] -> Bus Selector5/1
  Bus Selector4/1 -> MATLAB Function17/1(nmt_state)  "<NMT_state_4>"
  [HomingPosition_inc] -> Bus Selector9/1
  Bus Selector4/2 -> MATLAB Function19/1(mode)  "<mode_4>"
  MATLAB Function8/1(y) -> [stat2], Homing_m2/3(stat)
  [stat_mode_nmt_M3_M5_M6] -> Bus Selector4/1
  MATLAB Function9/1(y) -> Homing_m2/2(rx_mode)
  MATLAB Function2/1(y) -> [TargetReached_m2], Homing_m2/5(target_pos)
  Bus Selector3/2 -> MATLAB Function14/1(mode)  "<mode_3>"
  MATLAB Function13/1(y) -> [stat3], Homing_m3/3(stat)
  Bus Selector3/1 -> MATLAB Function12/1(nmt_state)  "<NMT_state_3>"
  Bus Selector11/1 -> Homing_m6/6(pos_ticks)  "<signal6>"
  [stat_mode_nmt_M3_M5_M6] -> Bus Selector2/1
  MATLAB Function14/1(y) -> Homing_m3/2(rx_mode)
  Bus Selector/2 -> MATLAB Function5/1(mode)  "<mode_1>"
  MATLAB Function3/1(y) -> Homing_m1/1(rx_nmt)
  [stat_mode_nmt_M3_M5_M6] -> Bus Selector3/1
  MATLAB Function15/1(y) -> Homing_m3/4(home_status)
  MATLAB Function19/1(y) -> Homing_m4/2(rx_mode)
  Bus Selector5/2 -> MATLAB Function29/1(mode)  "<mode_6>"
  Bus Selector5/1 -> MATLAB Function27/1(nmt_state)  "<NMT_state_6>"
  [HomingPosition_inc] -> Bus Selector7/1
  [HomingPosition_inc] -> Bus Selector6/1
  Bus Selector7/1 -> Homing_m2/6(pos_ticks)  "<signal2>"
  Bus Selector1/2 -> MATLAB Function9/1(mode)  "<mode_2>"
  Bus Selector2/2 -> MATLAB Function24/1(mode)  "<mode_5>"
  Homing_m6/1(Homing_status) -> [Homing_st6]  "status_6"
  Homing_m1/1(Homing_status) -> [Homing_st1]  "status_1"
  Homing_m2/1(Homing_status) -> [Homing_st2]  "status_2"
  Homing_m3/1(Homing_status) -> [Homing_st3]  "status_3"
  Homing_m5/1(Homing_status) -> [Homing_st5]  "status_5"
  Homing_m4/1(Homing_status) -> [Homing_st4]  "status_4"
  [Homing_st1] -> Sum/1
  [Homing_st2] -> Sum/2
  [Homing_st3] -> Sum/3
  [Homing_st4] -> Sum/4
  [Homing_st5] -> Sum/5
  [Homing_st6] -> Sum/6
  Sum/1 -> Compare To Constant/1
  Compare To Constant/1 -> Cast To Double/1
  Home_reference_inc/1 -> [HomingPosition_inc]
  [TargetReached_m1] -> Bus Creator/1  "m1"
  [TargetReached_m2] -> Bus Creator/2  "m2"
  [TargetReached_m3] -> Bus Creator/3  "m3"
  [TargetReached_m4] -> Bus Creator/4  "m4"
  [TargetReached_m5] -> Bus Creator/5  "m5"
  [TargetReached_m6] -> Bus Creator/6  "m6"
  Bus Creator/1 -> [TargetReached]
  Cast To Double/1 -> Homing_all_motors/1
  [stat1] -> MATLAB Function/1(stat1)
  [stat2] -> MATLAB Function/2(stat2)
  [stat3] -> MATLAB Function/3(stat3)
  [stat6] -> MATLAB Function/6(stat6)
  [stat4] -> MATLAB Function/4(stat4)
  [stat5] -> MATLAB Function/5(stat5)
  MATLAB Function/1(fault_error) -> [Fault_error]

== system ExoskeletonControlModel/DataProcessing/ShoulderFlexionImpedance ==
  Data Store Write10 : DataStoreWrite  DataStoreName=Spring_m5  IndexOptions=Index vector (dialog)  Indices=1  OutputSizes=1
  Data Store Write11 : DataStoreWrite  DataStoreName=Spring_m6  IndexOptions=Index vector (dialog)  Indices=1  OutputSizes=1
  Data Store Write12 : DataStoreWrite  DataStoreName=Damper_m5  IndexOptions=Index vector (dialog)  Indices=1  OutputSizes=1
  Data Store Write13 : DataStoreWrite  DataStoreName=Damper_m6  IndexOptions=Index vector (dialog)  Indices=1  OutputSizes=1
  Data Store Write14 : DataStoreWrite  DataStoreName=Damper_m1  IndexOptions=Index vector (dialog)  Indices=1  OutputSizes=1
  Data Store Write15 : DataStoreWrite  DataStoreName=Damper_m3  IndexOptions=Index vector (dialog)  Indices=1  OutputSizes=1
  Data Store Write16 : DataStoreWrite  DataStoreName=Damper_m2  IndexOptions=Index vector (dialog)  Indices=1  OutputSizes=1
  Data Store Write17 : DataStoreWrite  DataStoreName=Damper_m4  IndexOptions=Index vector (dialog)  Indices=1  OutputSizes=1
  Data Store Write6 : DataStoreWrite  DataStoreName=Spring_m1  IndexOptions=Index vector (dialog)  Indices=1  OutputSizes=1
  Data Store Write7 : DataStoreWrite  DataStoreName=Spring_m3  IndexOptions=Index vector (dialog)  Indices=1  OutputSizes=1
  Data Store Write8 : DataStoreWrite  DataStoreName=Spring_m2  IndexOptions=Index vector (dialog)  Indices=1  OutputSizes=1
  Data Store Write9 : DataStoreWrite  DataStoreName=Spring_m4  IndexOptions=Index vector (dialog)  Indices=1  OutputSizes=1
  d{1..6} (6 alike) : Constant  Value=0
  s{1..6} (6 alike) : Constant  Value=0
  wires:
  d3/1 -> Data Store Write15/1
  d2/1 -> Data Store Write16/1
  d1/1 -> Data Store Write14/1
  d5/1 -> Data Store Write12/1
  d6/1 -> Data Store Write13/1
  d4/1 -> Data Store Write17/1
  s5/1 -> Data Store Write10/1
  s4/1 -> Data Store Write9/1
  s3/1 -> Data Store Write7/1
  s2/1 -> Data Store Write8/1
  s6/1 -> Data Store Write11/1
  s1/1 -> Data Store Write6/1

== system ExoskeletonControlModel/DataProcessing/Subsystem ==
  note: END EFFECTOR ORIENTATION (WRIST) - RPY NOTATION
  note: HOMERUS ORIENTATION - RPY NOTATION
  sperical_pos1 : Inport
  Reset : Inport  Port=2
  ActualJointsConfigurations_rad : Inport  Port=3
  Enable : EnablePort
  Derivative : Derivative
  Derivative1 : Derivative
  Discrete-Time Integrator : DiscreteIntegrator  ExternalReset=rising  SampleTime=-1  ICPrevOutput=DiscIntNeverNeededParam  ICPrevScaledInput=DiscIntNeverNeededParam
  Discrete-Time Integrator1 : DiscreteIntegrator  ExternalReset=rising  SampleTime=-1  ICPrevOutput=DiscIntNeverNeededParam  ICPrevScaledInput=DiscIntNeverNeededParam
  Get Jacobian : robotmaniplib/Get Jacobian  RigidBodyTree=GiulioModel  EndEffector=body5  SimulateUsing=Interpreted execution
  Get Jacobian1 : robotmaniplib/Get Jacobian  RigidBodyTree=Giulio_Spheric_model  EndEffector=endeffector  SimulateUsing=Interpreted execution
  Get Transform : robotmaniplib/Get Transform  RigidBodyTree=GiulioModel  SourceBody=body5  TargetBody=base  SimulateUsing=Interpreted execution
  Get Transform1 : robotmaniplib/Get Transform  RigidBodyTree=GiulioModel  SourceBody=body5  TargetBody=base  SimulateUsing=Interpreted execution
  Get Transform2 : robotmaniplib/Get Transform  RigidBodyTree=Giulio_Spheric_model  SourceBody=endeffector  TargetBody=body0  SimulateUsing=Interpreted execution
  MATLAB Function : MATLAB Function  TreatAsAtomicUnit=on
  MATLAB Function1 : MATLAB Function  TreatAsAtomicUnit=on
  MATLAB Function2 : MATLAB Function  TreatAsAtomicUnit=on
  MATLAB Function3 : MATLAB Function  TreatAsAtomicUnit=on
  MATLAB Function4 : MATLAB Function  TreatAsAtomicUnit=on
  Mux : Mux  Inputs=3
  RPY_angles : slrealtimeloglib/File Log  decimation=1  inputProcessing=Elements as channels (sample based)
  RPY_spherical : slrealtimeloglib/File Log  decimation=1  inputProcessing=Elements as channels (sample based)
  XYZ : slrealtimeloglib/File Log  decimation=1  inputProcessing=Elements as channels (sample based)
  oriXYZ : slrealtimeloglib/File Log  decimation=1  inputProcessing=Elements as channels (sample based)
  spherical_joint_analitic_ori : slrealtimeloglib/File Log  decimation=1  inputProcessing=Elements as channels (sample based)
  actual_rpy : Outport
  wires:
  Reset/1 -> Discrete-Time Integrator1/2, Discrete-Time Integrator/2
  MATLAB Function4/1(y) -> Discrete-Time Integrator1/1
  Get Jacobian1/1 -> MATLAB Function4/1(u)
  MATLAB Function3/2(p) -> Mux/2  "pitch"
  Derivative/1 -> MATLAB Function4/2(x)
  Get Transform2/1 -> MATLAB Function3/1(u)
  Mux/1 -> actual_rpy/1, RPY_spherical/1
  MATLAB Function3/3(y) -> Mux/3  "yaw"
  sperical_pos1/1 -> Derivative/1, Get Jacobian1/1, Get Transform2/1
  Discrete-Time Integrator1/1 -> spherical_joint_analitic_ori/1
  MATLAB Function3/1(r) -> Mux/1  "roll"
  Discrete-Time Integrator/1 -> oriXYZ/1
  Get Transform1/1 -> MATLAB Function2/1(u)
  MATLAB Function2/1(y) -> RPY_angles/1
  MATLAB Function/1(y) -> XYZ/1
  ActualJointsConfigurations_rad/1 -> Get Transform1/1, Derivative1/1, Get Jacobian/1, Get Transform/1
  Derivative1/1 -> MATLAB Function1/2(x)
  Get Transform/1 -> MATLAB Function/1(u)
  Get Jacobian/1 -> MATLAB Function1/1(u)
  MATLAB Function1/1(y) -> Discrete-Time Integrator/1

== system ExoskeletonControlModel/DataProcessing/Subsystem1 ==
  WorkingChartState : Inport
  Constant1 : Constant  Value=0
  Delay1 : Delay  DelayLength=1
  MATLAB Function : MATLAB Function  TreatAsAtomicUnit=on
  Switch : Switch  Threshold=5  SaturateOnIntegerOverflow=off  InputSameDT=off
  Out1 : Outport
  wires:
  Constant1/1 -> Switch/3
  MATLAB Function/1(selectedEndedSignal) -> Switch/1
  Switch/1 -> Out1/1
  Delay1/1 -> MATLAB Function/1(WorkingState), Switch/2
  [signal_ended_el] -> MATLAB Function/3(EndedEL)
  [signal_ended_lr] -> MATLAB Function/4(EndedLR)
  [signal_ended_sh] -> MATLAB Function/2(EndedSH)
  WorkingChartState/1 -> Delay1/1

== system ExoskeletonControlModel/DataProcessing/Working_Chart/GoHome.GoHome_M1.ST1_set_PPM_M1 ==
  note: MOTOR 1 - MODE & INTERPOLATION TIME PERIOD
  Action Port : ActionPort
      settings: CopyFcn=Stateflow.SLINSF.SimulinkMan.removeBlockPreDeleteFcn  PreDeleteFcn=Stateflow.SLINSF.SimulinkMan.unsafePredeleteFcn
  Bus Creator3 : BusCreator  Inputs=2
  interpolation_period_m1 : Constant  Value=10
  mode_m1 : Constant
  receive_PDO2_m1 : Subsystem
  wires:
  Bus Creator3/1 -> receive_PDO2_m1/1(mode)
  mode_m1/1 -> Bus Creator3/1  "mode_m1"
  interpolation_period_m1/1 -> Bus Creator3/2  "interpolation_period_m1"

== system ExoskeletonControlModel/DataProcessing/Working_Chart/GoHome.GoHome_M1.ST2_Switch_on_Enable_M1 ==
  note: MOTOR 1 - CONTROLWORD
  Action Port : ActionPort
      settings: CopyFcn=Stateflow.SLINSF.SimulinkMan.removeBlockPreDeleteFcn  PreDeleteFcn=Stateflow.SLINSF.SimulinkMan.unsafePredeleteFcn
  controlword_m1 : Constant  Value=15
  receive_PDO1_m1 : Subsystem
  wires:
  controlword_m1/1 -> receive_PDO1_m1/1(controlword)

== system ExoskeletonControlModel/DataProcessing/Working_Chart/GoHome.GoHome_M1.ST3_send_target_pos_M1 ==
  note: MOTOR 1 - TARGET POSITION
  Action Port : ActionPort
      settings: CopyFcn=Stateflow.SLINSF.SimulinkMan.removeBlockPreDeleteFcn  PreDeleteFcn=Stateflow.SLINSF.SimulinkMan.unsafePredeleteFcn
  receive_PDO3_m1 : Subsystem
  target_position_m1 : Constant  Value=0
  wires:
  target_position_m1/1 -> receive_PDO3_m1/1(target_pos)

== system ExoskeletonControlModel/DataProcessing/Working_Chart/GoHome.GoHome_M1.ST4_Abs_ref_start_immediatly_M1 ==
  note: MOTOR 1 - CONTROLWORD
  Action Port : ActionPort
      settings: CopyFcn=Stateflow.SLINSF.SimulinkMan.removeBlockPreDeleteFcn  PreDeleteFcn=Stateflow.SLINSF.SimulinkMan.unsafePredeleteFcn
  controlword_m1 : Constant  Value=63
  receive_PDO1_m1 : Subsystem
  wires:
  controlword_m1/1 -> receive_PDO1_m1/1(controlword)

== system ExoskeletonControlModel/DataProcessing/Working_Chart/GoHome.GoHome_M2.ST1_set_PPM_M2 ==
  note: MOTOR 1 - MODE & INTERPOLATION TIME PERIOD
  Action Port : ActionPort
      settings: CopyFcn=Stateflow.SLINSF.SimulinkMan.removeBlockPreDeleteFcn  PreDeleteFcn=Stateflow.SLINSF.SimulinkMan.unsafePredeleteFcn
  Bus Creator3 : BusCreator  Inputs=2
  interpolation_period_m1 : Constant  Value=10
  mode_m1 : Constant
  receive_PDO2_m1 : Subsystem
  wires:
  Bus Creator3/1 -> receive_PDO2_m1/1(mode)
  mode_m1/1 -> Bus Creator3/1  "mode_m1"
  interpolation_period_m1/1 -> Bus Creator3/2  "interpolation_period_m1"

== system ExoskeletonControlModel/DataProcessing/Working_Chart/GoHome.GoHome_M2.ST2_Switch_on_Enable_M2 ==
  note: MOTOR 1 - CONTROLWORD
  Action Port : ActionPort
      settings: CopyFcn=Stateflow.SLINSF.SimulinkMan.removeBlockPreDeleteFcn  PreDeleteFcn=Stateflow.SLINSF.SimulinkMan.unsafePredeleteFcn
  controlword_m1 : Constant  Value=15
  receive_PDO1_m1 : Subsystem
  wires:
  controlword_m1/1 -> receive_PDO1_m1/1(controlword)

== system ExoskeletonControlModel/DataProcessing/Working_Chart/GoHome.GoHome_M2.ST3_send_target_pos_M2 ==
  note: MOTOR 1 - TARGET POSITION
  Action Port : ActionPort
      settings: CopyFcn=Stateflow.SLINSF.SimulinkMan.removeBlockPreDeleteFcn  PreDeleteFcn=Stateflow.SLINSF.SimulinkMan.unsafePredeleteFcn
  receive_PDO3_m1 : Subsystem
  target_position_m1 : Constant  Value=0
  wires:
  target_position_m1/1 -> receive_PDO3_m1/1(target_pos)

== system ExoskeletonControlModel/DataProcessing/Working_Chart/GoHome.GoHome_M2.ST4_Abs_ref_start_immediatly_M2 ==
  note: MOTOR 1 - CONTROLWORD
  Action Port : ActionPort
      settings: CopyFcn=Stateflow.SLINSF.SimulinkMan.removeBlockPreDeleteFcn  PreDeleteFcn=Stateflow.SLINSF.SimulinkMan.unsafePredeleteFcn
  controlword_m1 : Constant  Value=63
  receive_PDO1_m1 : Subsystem
  wires:
  controlword_m1/1 -> receive_PDO1_m1/1(controlword)

== system ExoskeletonControlModel/DataProcessing/Working_Chart/GoHome.GoHome_M3.ST1_set_PPM_M3 ==
  note: MOTOR 1 - MODE & INTERPOLATION TIME PERIOD
  Action Port : ActionPort
      settings: CopyFcn=Stateflow.SLINSF.SimulinkMan.removeBlockPreDeleteFcn  PreDeleteFcn=Stateflow.SLINSF.SimulinkMan.unsafePredeleteFcn
  Bus Creator3 : BusCreator  Inputs=2
  interpolation_period_m1 : Constant  Value=10
  mode_m1 : Constant
  receive_PDO2_m1 : Subsystem
  wires:
  Bus Creator3/1 -> receive_PDO2_m1/1(mode)
  mode_m1/1 -> Bus Creator3/1  "mode_m1"
  interpolation_period_m1/1 -> Bus Creator3/2  "interpolation_period_m1"

== system ExoskeletonControlModel/DataProcessing/Working_Chart/GoHome.GoHome_M3.ST2_Switch_on_Enable_M3 ==
  note: MOTOR 1 - CONTROLWORD
  Action Port : ActionPort
      settings: CopyFcn=Stateflow.SLINSF.SimulinkMan.removeBlockPreDeleteFcn  PreDeleteFcn=Stateflow.SLINSF.SimulinkMan.unsafePredeleteFcn
  controlword_m1 : Constant  Value=15
  receive_PDO1_m1 : Subsystem
  wires:
  controlword_m1/1 -> receive_PDO1_m1/1(controlword)

== system ExoskeletonControlModel/DataProcessing/Working_Chart/GoHome.GoHome_M3.ST3_send_target_pos_M3 ==
  note: MOTOR 1 - TARGET POSITION
  Action Port : ActionPort
      settings: CopyFcn=Stateflow.SLINSF.SimulinkMan.removeBlockPreDeleteFcn  PreDeleteFcn=Stateflow.SLINSF.SimulinkMan.unsafePredeleteFcn
  receive_PDO3_m1 : Subsystem
  target_position_m1 : Constant  Value=0
  wires:
  target_position_m1/1 -> receive_PDO3_m1/1(target_pos)

== system ExoskeletonControlModel/DataProcessing/Working_Chart/GoHome.GoHome_M3.ST4_Abs_ref_start_immediatly_M3 ==
  note: MOTOR 1 - CONTROLWORD
  Action Port : ActionPort
      settings: CopyFcn=Stateflow.SLINSF.SimulinkMan.removeBlockPreDeleteFcn  PreDeleteFcn=Stateflow.SLINSF.SimulinkMan.unsafePredeleteFcn
  controlword_m1 : Constant  Value=63
  receive_PDO1_m1 : Subsystem
  wires:
  controlword_m1/1 -> receive_PDO1_m1/1(controlword)

== system ExoskeletonControlModel/DataProcessing/Working_Chart/GoHome.GoHome_M4.ST1_set_PPM_M4 ==
  note: MOTOR 1 - MODE & INTERPOLATION TIME PERIOD
  Action Port : ActionPort
      settings: CopyFcn=Stateflow.SLINSF.SimulinkMan.removeBlockPreDeleteFcn  PreDeleteFcn=Stateflow.SLINSF.SimulinkMan.unsafePredeleteFcn
  Bus Creator3 : BusCreator  Inputs=2
  interpolation_period_m1 : Constant  Value=10
  mode_m1 : Constant
  receive_PDO2_m1 : Subsystem
  wires:
  Bus Creator3/1 -> receive_PDO2_m1/1(mode)
  mode_m1/1 -> Bus Creator3/1  "mode_m1"
  interpolation_period_m1/1 -> Bus Creator3/2  "interpolation_period_m1"

== system ExoskeletonControlModel/DataProcessing/Working_Chart/GoHome.GoHome_M4.ST2_Switch_on_Enable_M4 ==
  note: MOTOR 1 - CONTROLWORD
  Action Port : ActionPort
      settings: CopyFcn=Stateflow.SLINSF.SimulinkMan.removeBlockPreDeleteFcn  PreDeleteFcn=Stateflow.SLINSF.SimulinkMan.unsafePredeleteFcn
  controlword_m1 : Constant  Value=15
  receive_PDO1_m1 : Subsystem
  wires:
  controlword_m1/1 -> receive_PDO1_m1/1(controlword)
